simulink model "ComunicacionMATLABhomeIO_P4_meta"  (R2023b)
settings: Solver=VariableStepAuto  StartTime=0.0  StopTime=450000  RelTol=1e-3
values from neighbouring files (symbols this model uses):
  Ad = 0.991410640225    [mis_datos_completo.mat]    (also in mpc2.m = sysd.A)
  Bd = [0.000229789936787 7.39376207988e-05 0.000161351292089]    [mis_datos_completo.mat]    (also in mpc2.m = sysd.B)
  Cd = 89.7044193449    [mis_datos_completo.mat]    (also in mpc2.m = sysd.C)
  D = [0 0]    [mis_datos_completo.mat]    (also in mpc2.m = [0,0])
libraries: slpidlib x3, mpclib x2, simulink x1, realtime_pacer_lib x1
settings Model: Creator=usuario  LastModifiedBy=juanl_00e1ytj
settings SolverCC: AlgebraicLoopSolver=TrustRegion
settings DebuggingCC: UnconnectedInputMsg=warning  UnconnectedOutputMsg=warning  UnconnectedLineMsg=warning
settings ModelReferenceCC: EnableRefExpFcnMdlSchedulingChecks=on
settings RTWCC: DLArmComputeVersion=19.05

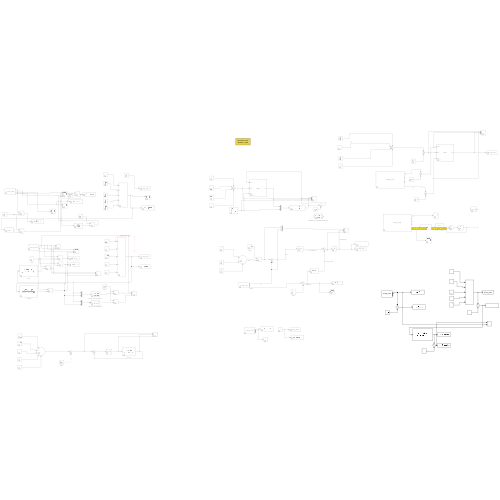
[thumbnail: Simulink's stored preview of the top-level diagram]
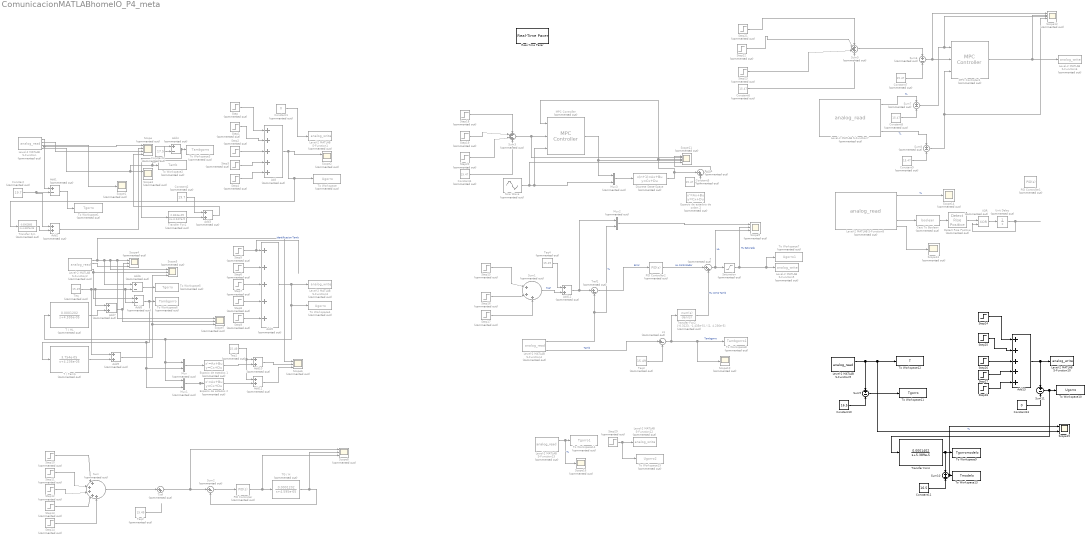
== system ComunicacionMATLABhomeIO_P4_meta ==
  Add : Sum  Commented=on  Inputs=+++++
  Add{1,4,6,8} (4 alike) : Sum  Commented=on  Inputs=+-
  Add{2..3,7,9..12} (7 alike) : Sum  Commented=on
  Add13 : Sum  Inputs=+++++
  Add5 : Sum  Commented=on  Inputs=+++++
  Cast To Boolean : DataTypeConversion  Commented=on  OutDataTypeStr=boolean  SaturateOnIntegerOverflow=off  RndMeth=Floor
  Constant : Constant  Commented=on  Value=19.7
  Constant1 : Constant  Commented=on  Value=0
  Constant10 : Constant  Value=16.5
  Constant11 : Constant  Value=16.5
  Constant13 : Constant  Value=0
  Constant2 : Constant  Commented=on  Value=19.7
  Constant3 : Constant  Commented=on  Value=17.5
  Constant{4..9} (6 alike) : Constant  Commented=on  Value=15.47
  Detect Rise Positive : simulink/Logic and Bit Operations/Detect Rise Positive  Commented=on  vinit=0  OutDataTypeStr=boolean
  Discrete State-Space : DiscreteStateSpace  Commented=on  A=Ad  B=Bd  C=Cd  D=D  SampleTime=-1
  Espacio de estadois de orden 2 : StateSpace  Commented=on  A=-3.866988642246605e-05  B=[-1.450262318829149e-06,-6.531519388547637e-07]  C=-71.051001498443750  D=[0,0]  InitialCondition=0
  Espacio de estados 1 : StateSpace  Commented=on  A=-3.866988642246605e-05  B=[-1.450262318829149e-06,-6.531519388547637e-07]  C=-71.051001498443750  D=[0,0]  InitialCondition=0
  Espacio de estados 2 : StateSpace  Commented=on  A=[-1.085279175702441e-05,-7.238690704198487e-06;2.846436093929025e-04,-1.013813759506818e-04]  B=[-6.619141197795110e-09,2.638251662156165e-07;-7.812195403938517e-06,8.332922523333637e-07]  C=[1.509873271789175e+02,0.349799874636245]  D=[0,0]  InitialCondition=0
  Level-2 MATLAB S-Function{,2,4,7..8,13} (6 alike) : M-S-Function  Commented=on  FunctionName=analog_read
  Level-2 MATLAB S-Function{1,3,5..6,12} (5 alike) : M-S-Function  Commented=on  FunctionName=analog_write
  Level-2 MATLAB S-Function10 : M-S-Function  FunctionName=analog_write
  Level-2 MATLAB S-Function9 : M-S-Function  FunctionName=analog_read
  MPC Controller : mpclib/MPC Controller  Commented=on  SCDEnableBlockLinearizationSpecification=on  mpcobj=MPCOBJ  is_multiple=0  enable_value=0  return_u0=off  updateMPCinCallerWorkspace=on  md_inport=on  mv_inport=off  uref_inport=off  return_cost=off  return_mvseq=off  return_qpstatus=off  return_xseq=off  return_state=off  return_ovseq=off  state_inport=off  umin_inport=off  umax_inport=off  ymin_inport=off  ymax_inport=off  cc_inport=off  ywt_inport=off  uwt_inport=off  duwt_inport=off  rhoeps_inport=off  pm_inport=off  MaximumP=10  HorizonChoice=FixedHorizon  n_ts=200  n_p=10  n_mv=1  n_md=1  n_ud=0  n_mo=1  n_uo=0  BlockDataType=double  SampleTimeInherited=off  switch_inport=off
  MPC Controller1 : mpclib/MPC Controller  Commented=on  SCDEnableBlockLinearizationSpecification=on  mpcobj=MPCOBJ  is_multiple=0  enable_value=0  return_u0=off  updateMPCinCallerWorkspace=on  md_inport=on  mv_inport=off  uref_inport=off  return_cost=off  return_mvseq=off  return_qpstatus=off  return_xseq=off  return_state=off  return_ovseq=off  state_inport=off  umin_inport=off  umax_inport=off  ymin_inport=off  ymax_inport=off  cc_inport=off  ywt_inport=off  uwt_inport=off  duwt_inport=off  rhoeps_inport=off  pm_inport=off  MaximumP=10  HorizonChoice=FixedHorizon  n_ts=200  n_p=10  n_mv=1  n_md=1  n_ud=0  n_mo=1  n_uo=0  BlockDataType=double  SampleTimeInherited=off  switch_inport=off
  Mux{,1..3} (4 alike) : Mux  Commented=on  Inputs=2
  PID Controller : slpidlib/PID Controller  Commented=on  Controller=PID  Form=Parallel  TimeDomain=Continuous-time  UseExternalTs=off  SampleTime=-1  IntegratorMethod=Forward Euler  FilterMethod=Forward Euler  ControllerParametersSource=internal  P=2.04826522870523  I=0.000214013083151844  UseKiTs=off  D=-1559.38300866482  N=0.000445239254280958  UseFilter=on  TunerSelectOption=Transfer Function Based (PID Tuner App)  InitialConditionSource=internal  InitialConditionForIntegrator=0  InitialConditionForFilter=0  DifferentiatorICPrevScaledInput=0  ExternalReset=none  TrackingMode=off  Kt=1  LimitOutput=off  SatLimitsSource=internal  UpperSaturationLimit=inf  LowerSaturationLimit=-inf  LinearizeAsGain=on  AntiWindupMode=none  Kb=1  LimitIntegrator=off  UpperIntegratorSaturationLimit=inf  LowerIntegratorSaturationLimit=-inf  POutMin=[]  POutMax=[]  IOutMin=[]  IOutMax=[]  DOutMin=[]  DOutMax=[]  NOutMin=[]  NOutMax=[]  SumOutMin=[]  SumOutMax=[]  SaturationOutMin=[]  SaturationOutMax=[]  PParamMin=[]  PParamMax=[]  IParamMin=[]  IParamMax=[]  DParamMin=[]  DParamMax=[]  NParamMin=[]  NParamMax=[]  KbParamMin=[]  KbParamMax=[]  KtParamMin=[]  KtParamMax=[]  KbOutMin=[]  KbOutMax=[]  KtOutMin=[]  KtOutMax=[]  IntegratorOutMin=[]  IntegratorOutMax=[]  FilterOutMin=[]  FilterOutMax=[]  SumI1OutMin=[]  SumI1OutMax=[]  SumI2OutMin=[]  SumI2OutMax=[]  SumI3OutMin=[]  SumI3OutMax=[]  SumI4OutMin=[]  SumI4OutMax=[]  SumDOutMin=[]  SumDOutMax=[]  DifferentiatorOutMin=[]  DifferentiatorOutMax=[]  FilterDiffOutCoefMin=[]  FilterDiffOutCoefMax=[]  ReciprocalOutMin=[]  ReciprocalOutMax=[]  SumDenOutMin=[]  SumDenOutMax=[]  SumNumOutMin=[]  SumNumOutMax=[]  DivideOutMin=[]  DivideOutMax=[]  UdiffTsProdOutMin=[]  UdiffTsProdOutMax=[]  NTsProdOutMin=[]  NTsProdOutMax=[]  UintegralTsProdOutMin=[]  UintegralTsProdOutMax=[]  UngainTsProdOutMin=[]  UngainTsProdOutMax=[]  ClampingZeroOutDataTypeStr=Inherit: Inherit via back propagation  ClampingZeroOutMin=[]  ClampingZeroOutMax=[]  FilterDenConstantOutDataTypeStr=Inherit: Inherit via back propagation  FilterDenConstantOutMin=[]  FilterDenConstantOutMax=[]  PCopyOutDataTypeStr=Inherit: Inherit via back propagation  PCopyOutMin=[]  PCopyOutMax=[]  NCopyOutDataTypeStr=Inherit: Inherit via back propagation  NCopyOutMin=[]  NCopyOutMax=[]  IntegratorContinuousStateAttributes=''  IntegratorStateMustResolveToSignalObject=off  IntegratorRTWStateStorageClass=Auto  FilterContinuousStateAttributes=''  FilterStateMustResolveToSignalObject=off  FilterRTWStateStorageClass=Auto  ParallelPVariant=InternalParameters  IdealPVariant=Disabled  IVariant=InternalParameters  DVariant=InternalParameters  IntegratorVariant=Continuous  SatVariant=Disabled  AWVariant=Passthrough  PCopyVariant=Disabled  TRVariant=Disabled  FdbkBlocksVariant=Forward  IdealPFdbkVariant=Disabled  SatFdbkVariant=Disabled  DerivativeFilterVariant=ContFilter  NVariant=InternalParameters  NCopyVariant=Disabled  FilterICVariant=InternalICsFilter  IntegratorICVariant=InternalICs  ExternalResetVariant=Disabled  TRSumVariant=Passthrough  SumFdbkVariant=Disabled  SumVariant=Sum_PID  TsampFilterVariant=InternalTs  TsampNgainVariant=Passthrough  TsampIntegralVariant=Disabled_SignalSpec  ExternalSaturationOutDataTypeStr=Inherit: Same as second input
  PID Controller1 : slpidlib/PID Controller  Commented=on  Controller=PID  Form=Parallel  TimeDomain=Continuous-time  UseExternalTs=off  SampleTime=-1  IntegratorMethod=Forward Euler  FilterMethod=Forward Euler  ControllerParametersSource=internal  P=0.511329579192054  I=4.69629397797088e-05  UseKiTs=off  D=-404.125554157073  N=0.000173734268901525  UseFilter=on  TunerSelectOption=Transfer Function Based (PID Tuner App)  InitialConditionSource=internal  InitialConditionForIntegrator=0  InitialConditionForFilter=0  DifferentiatorICPrevScaledInput=0  ExternalReset=none  TrackingMode=off  Kt=1  LimitOutput=off  SatLimitsSource=internal  UpperSaturationLimit=inf  LowerSaturationLimit=-inf  LinearizeAsGain=on  AntiWindupMode=none  Kb=1  LimitIntegrator=off  UpperIntegratorSaturationLimit=inf  LowerIntegratorSaturationLimit=-inf  POutMin=[]  POutMax=[]  IOutMin=[]  IOutMax=[]  DOutMin=[]  DOutMax=[]  NOutMin=[]  NOutMax=[]  SumOutMin=[]  SumOutMax=[]  SaturationOutMin=[]  SaturationOutMax=[]  PParamMin=[]  PParamMax=[]  IParamMin=[]  IParamMax=[]  DParamMin=[]  DParamMax=[]  NParamMin=[]  NParamMax=[]  KbParamMin=[]  KbParamMax=[]  KtParamMin=[]  KtParamMax=[]  KbOutMin=[]  KbOutMax=[]  KtOutMin=[]  KtOutMax=[]  IntegratorOutMin=[]  IntegratorOutMax=[]  FilterOutMin=[]  FilterOutMax=[]  SumI1OutMin=[]  SumI1OutMax=[]  SumI2OutMin=[]  SumI2OutMax=[]  SumI3OutMin=[]  SumI3OutMax=[]  SumI4OutMin=[]  SumI4OutMax=[]  SumDOutMin=[]  SumDOutMax=[]  DifferentiatorOutMin=[]  DifferentiatorOutMax=[]  FilterDiffOutCoefMin=[]  FilterDiffOutCoefMax=[]  ReciprocalOutMin=[]  ReciprocalOutMax=[]  SumDenOutMin=[]  SumDenOutMax=[]  SumNumOutMin=[]  SumNumOutMax=[]  DivideOutMin=[]  DivideOutMax=[]  UdiffTsProdOutMin=[]  UdiffTsProdOutMax=[]  NTsProdOutMin=[]  NTsProdOutMax=[]  UintegralTsProdOutMin=[]  UintegralTsProdOutMax=[]  UngainTsProdOutMin=[]  UngainTsProdOutMax=[]  ClampingZeroOutDataTypeStr=Inherit: Inherit via back propagation  ClampingZeroOutMin=[]  ClampingZeroOutMax=[]  FilterDenConstantOutDataTypeStr=Inherit: Inherit via back propagation  FilterDenConstantOutMin=[]  FilterDenConstantOutMax=[]  PCopyOutDataTypeStr=Inherit: Inherit via back propagation  PCopyOutMin=[]  PCopyOutMax=[]  NCopyOutDataTypeStr=Inherit: Inherit via back propagation  NCopyOutMin=[]  NCopyOutMax=[]  IntegratorContinuousStateAttributes=''  IntegratorStateMustResolveToSignalObject=off  IntegratorRTWStateStorageClass=Auto  FilterContinuousStateAttributes=''  FilterStateMustResolveToSignalObject=off  FilterRTWStateStorageClass=Auto  ParallelPVariant=InternalParameters  IdealPVariant=Disabled  IVariant=InternalParameters  DVariant=InternalParameters  IntegratorVariant=Continuous  SatVariant=Disabled  AWVariant=Passthrough  PCopyVariant=Disabled  TRVariant=Disabled  FdbkBlocksVariant=Forward  IdealPFdbkVariant=Disabled  SatFdbkVariant=Disabled  DerivativeFilterVariant=ContFilter  NVariant=InternalParameters  NCopyVariant=Disabled  FilterICVariant=InternalICsFilter  IntegratorICVariant=InternalICs  ExternalResetVariant=Disabled  TRSumVariant=Passthrough  SumFdbkVariant=Disabled  SumVariant=Sum_PID  TsampFilterVariant=InternalTs  TsampNgainVariant=Passthrough  TsampIntegralVariant=Disabled_SignalSpec  ExternalSaturationOutDataTypeStr=Inherit: Same as second input
  PID Controller2 : slpidlib/PID Controller  Commented=on  Controller=PID  Form=Parallel  TimeDomain=Continuous-time  UseExternalTs=off  SampleTime=-1  IntegratorMethod=Forward Euler  FilterMethod=Forward Euler  ControllerParametersSource=internal  P=2.04826522870523  I=0.000214013083151844  UseKiTs=off  D=-1559.38300866482  N=0.000445239254280958  UseFilter=on  TunerSelectOption=Transfer Function Based (PID Tuner App)  InitialConditionSource=internal  InitialConditionForIntegrator=0  InitialConditionForFilter=0  DifferentiatorICPrevScaledInput=0  ExternalReset=none  TrackingMode=off  Kt=1  LimitOutput=off  SatLimitsSource=internal  UpperSaturationLimit=inf  LowerSaturationLimit=-inf  LinearizeAsGain=on  AntiWindupMode=none  Kb=1  LimitIntegrator=off  UpperIntegratorSaturationLimit=inf  LowerIntegratorSaturationLimit=-inf  POutMin=[]  POutMax=[]  IOutMin=[]  IOutMax=[]  DOutMin=[]  DOutMax=[]  NOutMin=[]  NOutMax=[]  SumOutMin=[]  SumOutMax=[]  SaturationOutMin=[]  SaturationOutMax=[]  PParamMin=[]  PParamMax=[]  IParamMin=[]  IParamMax=[]  DParamMin=[]  DParamMax=[]  NParamMin=[]  NParamMax=[]  KbParamMin=[]  KbParamMax=[]  KtParamMin=[]  KtParamMax=[]  KbOutMin=[]  KbOutMax=[]  KtOutMin=[]  KtOutMax=[]  IntegratorOutMin=[]  IntegratorOutMax=[]  FilterOutMin=[]  FilterOutMax=[]  SumI1OutMin=[]  SumI1OutMax=[]  SumI2OutMin=[]  SumI2OutMax=[]  SumI3OutMin=[]  SumI3OutMax=[]  SumI4OutMin=[]  SumI4OutMax=[]  SumDOutMin=[]  SumDOutMax=[]  DifferentiatorOutMin=[]  DifferentiatorOutMax=[]  FilterDiffOutCoefMin=[]  FilterDiffOutCoefMax=[]  ReciprocalOutMin=[]  ReciprocalOutMax=[]  SumDenOutMin=[]  SumDenOutMax=[]  SumNumOutMin=[]  SumNumOutMax=[]  DivideOutMin=[]  DivideOutMax=[]  UdiffTsProdOutMin=[]  UdiffTsProdOutMax=[]  NTsProdOutMin=[]  NTsProdOutMax=[]  UintegralTsProdOutMin=[]  UintegralTsProdOutMax=[]  UngainTsProdOutMin=[]  UngainTsProdOutMax=[]  ClampingZeroOutDataTypeStr=Inherit: Inherit via back propagation  ClampingZeroOutMin=[]  ClampingZeroOutMax=[]  FilterDenConstantOutDataTypeStr=Inherit: Inherit via back propagation  FilterDenConstantOutMin=[]  FilterDenConstantOutMax=[]  PCopyOutDataTypeStr=Inherit: Inherit via back propagation  PCopyOutMin=[]  PCopyOutMax=[]  NCopyOutDataTypeStr=Inherit: Inherit via back propagation  NCopyOutMin=[]  NCopyOutMax=[]  IntegratorContinuousStateAttributes=''  IntegratorStateMustResolveToSignalObject=off  IntegratorRTWStateStorageClass=Auto  FilterContinuousStateAttributes=''  FilterStateMustResolveToSignalObject=off  FilterRTWStateStorageClass=Auto  ParallelPVariant=InternalParameters  IdealPVariant=Disabled  IVariant=InternalParameters  DVariant=InternalParameters  IntegratorVariant=Continuous  SatVariant=Disabled  AWVariant=Passthrough  PCopyVariant=Disabled  TRVariant=Disabled  FdbkBlocksVariant=Forward  IdealPFdbkVariant=Disabled  SatFdbkVariant=Disabled  DerivativeFilterVariant=ContFilter  NVariant=InternalParameters  NCopyVariant=Disabled  FilterICVariant=InternalICsFilter  IntegratorICVariant=InternalICs  ExternalResetVariant=Disabled  TRSumVariant=Passthrough  SumFdbkVariant=Disabled  SumVariant=Sum_PID  TsampFilterVariant=InternalTs  TsampNgainVariant=Passthrough  TsampIntegralVariant=Disabled_SignalSpec  ExternalSaturationOutDataTypeStr=Inherit: Same as second input
  Real-Time Pacer : realtime_pacer_lib/Real-Time Pacer  simTimePerRealTime=5000
      settings: SourceProductName=Real-Time Pacer
  Saturation : Saturate  Commented=on  UpperLimit=50e20  LowerLimit=0
  Scope : Scope  Commented=on  NumInputPorts=4
  Scope{1,10,13..14,16} (5 alike) : Scope  Commented=on
  Scope11 : Scope  Commented=on  NumInputPorts=5
  Scope12 : Scope  Commented=on  NumInputPorts=5
  Scope15 : Scope  NumInputPorts=2
  Scope2 : Scope  Commented=on  NumInputPorts=2
  Scope{3..9} (7 alike) : Scope  Commented=on  NumInputPorts=3
  Sine Wave : Sin  Commented=on  Amplitude=7  Bias=15.47  Frequency=72.65e-6  SampleTime=0
  Step{,5,15,18,29} (5 alike) : Step  Commented=on  Time=0  After=0  SampleTime=0
  Step1 : Step  Commented=on  Time=20000  SampleTime=0
  Step10 : Step  Commented=on  Time=0  Before=2  After=0  SampleTime=0
  Step11 : Step  Commented=on  Time=50000  After=3  SampleTime=0
  Step12 : Step  Commented=on  Time=85000  SampleTime=0
  Step13 : Step  Commented=on  Time=190000  Before=2  After=0  SampleTime=0
  Step14 : Step  Commented=on  Time=300000  After=3  SampleTime=0
  Step16 : Step  Commented=on  Time=160000  After=12  SampleTime=0
  Step17 : Step  Commented=on  Time=300000  After=-6  SampleTime=0
  Step19 : Step  Commented=on  Time=160000  After=12  SampleTime=0
  Step2 : Step  Commented=on  Time=85000  After=2  SampleTime=0
  Step20 : Step  Commented=on  Time=300000  After=-6  SampleTime=0
  Step21 : Step  Commented=on  Time=0  After=5  SampleTime=0
  Step22 : Step  Commented=on  Time=160000  After=7  SampleTime=0
  Step23 : Step  Commented=on  Time=300000  After=-6  SampleTime=0
  Step24 : Step  Time=0  After=0  SampleTime=0
  Step25 : Step  Time=50000  After=2  SampleTime=0
  Step26 : Step  Time=125000  After=2  SampleTime=0
  Step27 : Step  Time=230000  After=2  SampleTime=0
  Step28 : Step  Time=350000  After=3  SampleTime=0
  Step3 : Step  Commented=on  Time=190000  After=3  SampleTime=0
  Step4 : Step  Commented=on  Time=300000  After=3  SampleTime=0
  Step6 : Step  Commented=on  Time=20000  SampleTime=0
  Step7 : Step  Commented=on  Time=85000  After=2  SampleTime=0
  Step8 : Step  Commented=on  Time=190000  After=3  SampleTime=0
  Step9 : Step  Commented=on  Time=300000  After=3  SampleTime=0
  Sum : Sum  Commented=on  Inputs=|+++++
  Sum1 : Sum  Commented=on  Inputs=|+++
  Sum10 : Sum  Inputs=+|+
  Sum11 : Sum  Inputs=+|-
  Sum2 : Sum  Commented=on  Inputs=|+-
  Sum3 : Sum  Commented=on  Inputs=++++
  Sum4 : Sum  Commented=on  Inputs=|++
  Sum5 : Sum  Commented=on  Inputs=++++
  Sum6 : Sum  Commented=on  Inputs=+|-
  Sum7 : Sum  Commented=on  Inputs=+|-
  Sum8 : Sum  Commented=on  Inputs=+|-
  Sum9 : Sum  Inputs=+|-
  T / HL : TransferFcn  Commented=on  Numerator=[0.0001202]  Denominator=[1 4.595e-05]
  T / Tamb : TransferFcn  Commented=on  Numerator=[3.754e-05]  Denominator=[1 4.236e-05]
  TG / H : TransferFcn  Commented=on  Numerator=[0.0001202]  Denominator=[1 4.595e-05]
  Teq{,1..4} (5 alike) : Constant  Commented=on  Value=15.49
  To Workspace : ToWorkspace  Commented=on  VariableName=Ugorro  SampleTime=-1
  To Workspace1 : ToWorkspace  Commented=on  VariableName=Tgorro  SampleTime=-1
  To Workspace10 : ToWorkspace  VariableName=Ugorro  SampleTime=-1
  To Workspace11 : ToWorkspace  VariableName=Tgorro  SampleTime=-1
  To Workspace12 : ToWorkspace  VariableName=T  SampleTime=-1
  To Workspace13 : ToWorkspace  VariableName=Tmodelo  SampleTime=-1
  To Workspace14 : ToWorkspace  Commented=on  VariableName=Tgorro1  SampleTime=-1
  To Workspace15 : ToWorkspace  Commented=on  VariableName=Ugorro2  SampleTime=-1
  To Workspace2 : ToWorkspace  Commented=on  VariableName=Tamb  SampleTime=-1
  To Workspace3 : ToWorkspace  Commented=on  VariableName=Tambgorro  SampleTime=-1
  To Workspace4 : ToWorkspace  Commented=on  VariableName=Ugorro  SampleTime=-1
  To Workspace5 : ToWorkspace  Commented=on  VariableName=Tgorro  SampleTime=-1
  To Workspace6 : ToWorkspace  Commented=on  VariableName=Tambgorro  SampleTime=-1
  To Workspace7 : ToWorkspace  Commented=on  VariableName=Ugorro1  SampleTime=-1
  To Workspace8 : ToWorkspace  Commented=on  VariableName=Tambgorro1  SampleTime=-1
  To Workspace9 : ToWorkspace  VariableName=Tgorromodelo  SampleTime=-1
  Transfer Fcn : TransferFcn  Commented=on  Numerator=[0.0002893]  Denominator=[1 4.597e-05]
  Transfer Fcn1 : TransferFcn  Commented=on  Numerator=[2.843e-05]  Denominator=[1 4.247e-5]
  Transfer Fcn2 : TransferFcn  Commented=on  Numerator=[-0.3123, -1.435e-5]  Denominator=[1, 4.236e-5]
  Transfer Fcn4 : TransferFcn  Numerator=[0.0001402]  Denominator=[1 5.389e-5]
  Tref : Sum  Commented=on  Inputs=|++
  Tref1 : Sum  Commented=on  Inputs=|+-
  Unit Delay : UnitDelay  Commented=on  SampleTime=-1  HasFrameUpgradeWarning=on
  XOR : Logic  Commented=on  Operator=XOR  IconShape=distinctive  AllPortsSameDT=off  OutDataTypeStr=boolean
  s : Sum  Commented=on  Inputs=|++
  s1 : Sum  Commented=on  Inputs=|+-
  wires:
  Level-2 MATLAB S-Function/1 -> Scope/1, Add1/1
  Step/1 -> Add/1
  Add/1 -> Transfer Fcn/1, To Workspace/1, Scope2/1
  Step1/1 -> Add/2
  Level-2 MATLAB S-Function/3 -> Scope1/1
  Level-2 MATLAB S-Function/2 -> Scope/3
  Step4/1 -> Add/5
  Step3/1 -> Add/4
  Step2/1 -> Add/3
  Constant/1 -> Add2/1, Add1/2
  Add1/1 -> To Workspace1/1
  Transfer Fcn/1 -> Add2/2
  Add2/1 -> Scope/2
  Level-2 MATLAB S-Function/4 -> Add4/1, To Workspace2/1, Scope3/1
  Constant1/1 -> Level-2 MATLAB S-Function1/1
  Constant2/1 -> Add3/1
  Transfer Fcn1/1 -> Add3/2
  Add3/1 -> Scope/4
  Add4/1 -> Transfer Fcn1/1, To Workspace3/1
  Constant3/1 -> Add4/2
  Level-2 MATLAB S-Function2/1 -> Scope6/1, Scope5/1, Scope7/1, Scope4/1, Add6/1
  Level-2 MATLAB S-Function2/2 -> Scope4/3
  Step5/1 -> Add5/1  "Identificacion Tamb"
  Step6/1 -> Add5/2
  Step7/1 -> Add5/3
  Step9/1 -> Add5/5
  Step8/1 -> Add5/4
  Teq/1 -> Add9/1, Add7/1, Add8/2, Add6/2
  Add6/1 -> To Workspace5/1
  T / HL/1 -> Add7/2
  Add7/1 -> Scope7/2, Scope4/2
  Level-2 MATLAB S-Function2/4 -> Add8/1, Scope5/2
  T / Tamb/1 -> Add9/2
  Add9/1 -> Scope7/3, Scope5/3
  Mux/1 -> Espacio de estados 1/1
  Teq1/1 -> Add11/1, Add10/1
  Espacio de estados 1/1 -> Add10/2
  Add10/1 -> Scope6/2
  Add5/1 -> Level-2 MATLAB S-Function3/1, Mux/1, Mux1/1, T / HL/1, To Workspace4/1
  Add8/1 -> Mux1/2, Mux/2, T / Tamb/1, To Workspace6/1
  Mux1/1 -> Espacio de estados 2/1
  Espacio de estados 2/1 -> Add11/2
  Add11/1 -> Scope6/3
  Teq2/1 -> ?
  Step10/1 -> Sum/1
  Sum/1 -> Tref/1
  Sum2/1 -> PID Controller/1
  Tref/1 -> Scope8/1, Sum2/1
  Step11/1 -> Sum/2
  PID Controller/1 -> Scope8/3, TG / H/1
  Step13/1 -> Sum/4
  Step12/1 -> Sum/3
  TG / H/1 -> Scope8/2, Sum2/2
  Step14/1 -> Sum/5
  Step16/1 -> Sum1/2
  Step15/1 -> Sum1/1
  Step17/1 -> Sum1/3
  Level-2 MATLAB S-Function4/1 -> Mux2/2, Tref1/2  "TL"
  Level-2 MATLAB S-Function4/4 -> s1/1  "Tamb"
  Tref1/1 -> PID Controller2/1  "Error"
  PID Controller2/1 -> s/1  "HL Controlador"
  s/1 -> Scope9/3, Saturation/1  "HL"
  Mux2/1 -> Scope9/1
  Transfer Fcn2/1 -> s/2  "HL comp Tamb"
  Teq3/1 -> s1/2
  s1/1 -> Transfer Fcn2/1, Scope10/1, To Workspace8/1  "Tambgorro"
  Sum1/1 -> Add12/2  "Tref"
  Teq4/1 -> Add12/1
  Add12/1 -> Mux2/1, Tref1/1
  Saturation/1 -> Scope9/2, To Workspace7/1, Level-2 MATLAB S-Function5/1  "HL Saturada"
  Step18/1 -> Sum3/1
  Step20/1 -> Sum3/3
  Step19/1 -> Sum3/2
  Sum3/1 -> Scope11/2, MPC Controller/2
  Mux3/1 -> Discrete State-Space/1
  MPC Controller/1 -> Scope11/4, Mux3/1
  Sine Wave/1 -> Scope11/5, MPC Controller/3, Mux3/2
  Constant4/1 -> Sum3/4
  Discrete State-Space/1 -> Sum4/1, MPC Controller/1, Scope11/3
  Constant5/1 -> Sum4/2
  Sum4/1 -> Scope11/1
  Constant6/1 -> Sum5/4
  Step22/1 -> Sum5/2
  Step23/1 -> Sum5/3
  Step21/1 -> Sum5/1
  Sum5/1 -> Sum6/1
  Constant7/1 -> Sum6/2
  Sum6/1 -> Scope12/1, MPC Controller1/2
  MPC Controller1/1 -> Scope12/2, Level-2 MATLAB S-Function6/1
  Level-2 MATLAB S-Function7/1 -> Sum7/1  "TL"
  Constant8/1 -> Sum7/2
  Sum7/1 -> Scope12/3, MPC Controller1/1
  Sum8/1 -> Scope12/4, MPC Controller1/3
  Constant9/1 -> Sum8/2
  Level-2 MATLAB S-Function7/4 -> Sum8/1  "TL"
  Level-2 MATLAB S-Function8/5 -> Cast To Boolean/1
  Cast To Boolean/1 -> Detect Rise Positive/1
  Detect Rise Positive/1 -> XOR/1
  XOR/1 -> Unit Delay/1
  Unit Delay/1 -> XOR/2
  Level-2 MATLAB S-Function8/6 -> Scope13/1
  Level-2 MATLAB S-Function8/1 -> Scope14/1  "TL"
  Level-2 MATLAB S-Function9/1 -> Sum9/1, Scope15/2, To Workspace12/1  "TL"
  Step27/1 -> Add13/4
  Step28/1 -> Add13/5
  Step25/1 -> Add13/2
  Step24/1 -> Add13/1
  Step26/1 -> Add13/3
  Constant10/1 -> Sum9/2
  Sum9/1 -> To Workspace11/1
  Transfer Fcn4/1 -> To Workspace9/1, Sum10/1
  Sum10/1 -> Scope15/1, To Workspace13/1
  Constant11/1 -> Sum10/2
  Add13/1 -> Sum11/1, Level-2 MATLAB S-Function10/1
  Constant13/1 -> Sum11/2
  Sum11/1 -> Transfer Fcn4/1, To Workspace10/1
  Step29/1 -> To Workspace15/1, Level-2 MATLAB S-Function12/1
  Level-2 MATLAB S-Function13/1 -> Scope16/1, To Workspace14/1  "TL"
